simulink model "experiment"  (R2021b)
settings: Solver=VariableStepAuto  StartTime=0.0  StopTime=40  FixedStep=1  RelTol=1e-3
InitFcn:
  | InitFcn;
StopFcn:
  | PostFunction;
values from neighbouring files (symbols this model uses):
  desiredSpeed = -10    [InitFcn.m]
  LookDistance = 0.4    [InitFcn.m]
  vehicleDynamics = [b1 L1 L2 b2]    [InitFcn.m]
  X_waypoints = [X_waypoints, linspace(L1-L2-R1, L1-L2-R1, n)]    [InitFcn.m]
  Y_waypoints = [Y_waypoints, linspace(-R1,-R1-L3,n)]    [InitFcn.m]
undefined symbols (not defined in the file or in its folder): Index, X_waypoints_2, Y_waypoints_2
libraries: slpidlib x1
settings Model: Creator=juliu  LastModifiedBy=marti
settings SolverCC: AlgebraicLoopSolver=TrustRegion
settings DataIOCC: SaveFormat=StructureWithTime  ReturnWorkspaceOutputs=off
settings OptimizationCC: BlockReduction=off  BufferReuse=off
settings DebuggingCC: AlgebraicLoopMsg=none  UnconnectedInputMsg=none  UnconnectedOutputMsg=none  UnconnectedLineMsg=none  SFMachineParentedDataDiag=warning

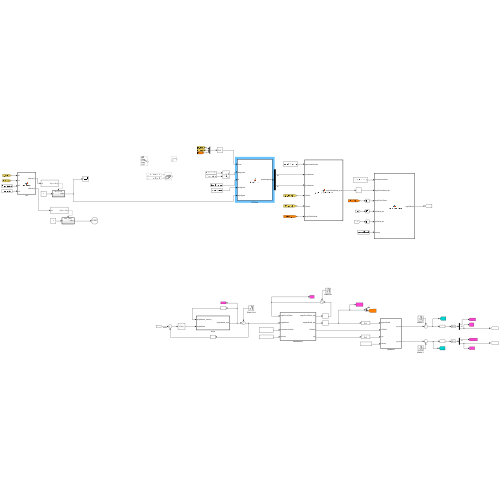
[thumbnail: Simulink's stored preview of the top-level diagram]
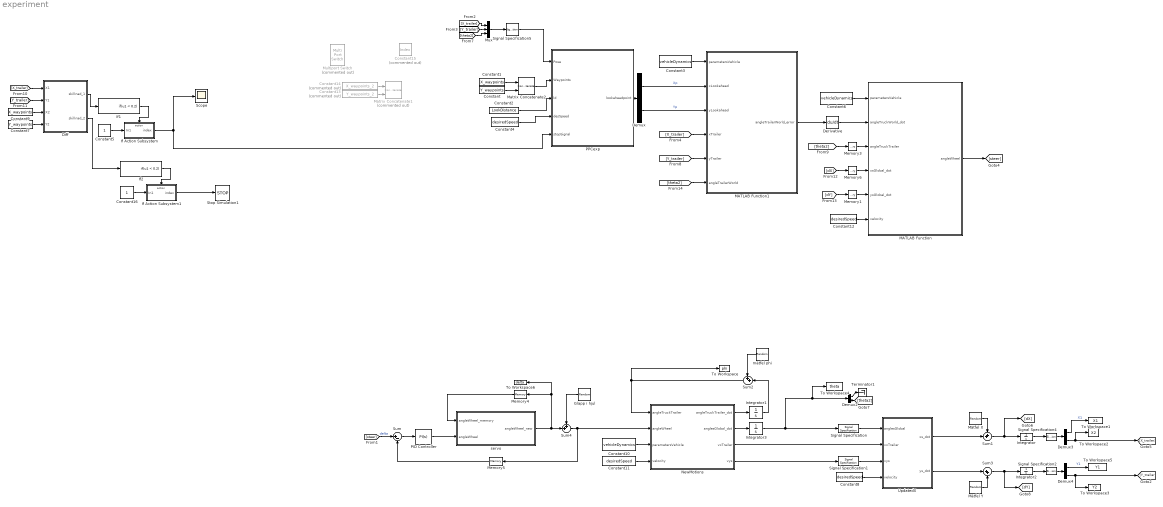
== system experiment ==
  Constant : Constant  Value=Y_waypoints
  Constant1 : Constant  Value=X_waypoints
  Constant10 : Constant  Value=vehicleDynamics
  Constant{4,8,11..12} (4 alike) : Constant  Value=desiredSpeed
  Constant13 : Constant  Commented=on  Value=Y_waypoints_2
  Constant14 : Constant  Commented=on  Value=X_waypoints_2
  Constant15 : Constant  Commented=on  Value=Index
  Constant16 : Constant
  Constant2 : Constant  Value=LookDistance
  Constant3 : Constant  Value=vehicleDynamics
  Constant5 : Constant
  Constant6 : Constant  Value=vehicleDynamics
  Constant7 : Constant  Value=Y_waypoints
  Constant9 : Constant  Value=X_waypoints
  Demux{,2..4} (4 alike) : Demux  Outputs=2
  Derivative : Derivative
  Diff : MATLAB Function  TreatAsAtomicUnit=on
  Glapp i hjul : RandomNumber  Variance=(pi/360)^2  SampleTime=3
  If Action Subsystem : Subsystem  TreatAsAtomicUnit=on
  If Action Subsystem1 : Subsystem  TreatAsAtomicUnit=on
  If1 : If  IfExpression=u1 < 0.2  ShowElse=off
  If2 : If  IfExpression=u1 < 0.2  ShowElse=off
  Integrator : Integrator  InitialCondition=[0;-1.3]
  Integrator1 : Integrator
  Integrator2 : Integrator
  Integrator3 : Integrator
  MATLAB Function : MATLAB Function  TreatAsAtomicUnit=on
  MATLAB Function1 : MATLAB Function  TreatAsAtomicUnit=on
  Matrix Concatenate1 : Concatenate  Commented=on  Mode=Multidimensional array  ConcatenateDimension=2
  Matrix Concatenate2 : Concatenate  Mode=Multidimensional array  ConcatenateDimension=2
  Memory{1,3..6} (5 alike) : Memory
  Multiport Switch : MultiPortSwitch  Commented=on
  Mux : Mux  Inputs=3
  Mätfel X : RandomNumber  Variance=(4e-5)^2  SampleTime=0.1
  Mätfel Y : RandomNumber  Variance=(4e-5)^2  SampleTime=0.1
  NewMotions : MATLAB Function  TreatAsAtomicUnit=on
  PID Controller : slpidlib/PID Controller  Controller=PI  Form=Parallel  TimeDomain=Continuous-time  UseExternalTs=off  SampleTime=-1  IntegratorMethod=Forward Euler  FilterMethod=Forward Euler  ControllerParametersSource=internal  P=2.10  I=0.50  D=0  UseFilter=on  N=100  TunerSelectOption=Transfer Function Based (PID Tuner App)  InitialConditionSource=internal  InitialConditionForIntegrator=0  InitialConditionForFilter=0  DifferentiatorICPrevScaledInput=0  ExternalReset=none  TrackingMode=off  Kt=1  LimitOutput=off  SatLimitsSource=internal  UpperSaturationLimit=inf  LowerSaturationLimit=-inf  LinearizeAsGain=on  AntiWindupMode=none  Kb=1  POutMin=[]  POutMax=[]  IOutMin=[]  IOutMax=[]  DOutMin=[]  DOutMax=[]  NOutMin=[]  NOutMax=[]  SumOutMin=[]  SumOutMax=[]  SaturationOutMin=[]  SaturationOutMax=[]  PParamMin=[]  PParamMax=[]  IParamMin=[]  IParamMax=[]  DParamMin=[]  DParamMax=[]  NParamMin=[]  NParamMax=[]  KbParamMin=[]  KbParamMax=[]  KtParamMin=[]  KtParamMax=[]  KbOutMin=[]  KbOutMax=[]  KtOutMin=[]  KtOutMax=[]  IntegratorOutMin=[]  IntegratorOutMax=[]  FilterOutMin=[]  FilterOutMax=[]  SumI1OutMin=[]  SumI1OutMax=[]  SumI2OutMin=[]  SumI2OutMax=[]  SumI3OutMin=[]  SumI3OutMax=[]  SumI4OutMin=[]  SumI4OutMax=[]  SumDOutMin=[]  SumDOutMax=[]  DifferentiatorOutMin=[]  DifferentiatorOutMax=[]  FilterDiffOutCoefMin=[]  FilterDiffOutCoefMax=[]  ReciprocalOutMin=[]  ReciprocalOutMax=[]  SumDenOutMin=[]  SumDenOutMax=[]  SumNumOutMin=[]  SumNumOutMax=[]  DivideOutMin=[]  DivideOutMax=[]  UdiffTsProdOutMin=[]  UdiffTsProdOutMax=[]  NTsProdOutMin=[]  NTsProdOutMax=[]  UintegralTsProdOutMin=[]  UintegralTsProdOutMax=[]  UngainTsProdOutMin=[]  UngainTsProdOutMax=[]  IntegratorContinuousStateAttributes=''  IntegratorStateMustResolveToSignalObject=off  IntegratorRTWStateStorageClass=Auto  FilterContinuousStateAttributes=''  FilterStateMustResolveToSignalObject=off  FilterRTWStateStorageClass=Auto  ParallelPVariant=InternalParameters  IdealPVariant=Disabled  IVariant=InternalParameters  DVariant=Disabled  IntegratorVariant=Continuous  SatVariant=Disabled  AWVariant=Passthrough  PCopyVariant=Disabled  TRVariant=Disabled  FdbkBlocksVariant=Forward  IdealPFdbkVariant=Disabled  SatFdbkVariant=Disabled  DerivativeFilterVariant=Disabled  NVariant=Disabled  NCopyVariant=Disabled_SignalSpec  FilterICVariant=Disabled  IntegratorICVariant=InternalICs  ExternalResetVariant=Disabled  TRSumVariant=Passthrough  SumFdbkVariant=Disabled  SumVariant=Sum_PI  TsampFilterVariant=InternalTs  TsampNgainVariant=Passthrough  TsampIntegralVariant=Passthrough  ExternalSaturationOutDataTypeStr=Inherit: Same as second input
  PPCexp : MATLAB Function  TreatAsAtomicUnit=on
  Scope : Scope
  Signal Specification{,1..2,4} (4 alike) : SignalSpecification  Dimensions=2
  Signal Specification5 : SignalSpecification  Dimensions=3
  Stop Simulation1 : Stop
  Sum : Sum  Inputs=|+-
  Sum1 : Sum  Inputs=++|
  Sum2 : Sum  Inputs=++|
  Sum3 : Sum  Inputs=|++
  Sum4 : Sum  Inputs=++|
  Terminator1 : Terminator
  To Workspace : ToWorkspace  VariableName=phi  SampleTime=-1
  To Workspace1 : ToWorkspace  VariableName=X1  SampleTime=-1
  To Workspace2 : ToWorkspace  VariableName=X2  SampleTime=-1
  To Workspace3 : ToWorkspace  VariableName=Y2  SampleTime=-1
  To Workspace4 : ToWorkspace  VariableName=theta  SampleTime=-1
  To Workspace5 : ToWorkspace  VariableName=Y1  SampleTime=-1
  To Workspace6 : ToWorkspace  VariableName=delta  SampleTime=-1
  UpdatedX : MATLAB Function  TreatAsAtomicUnit=on
  mätfel phi : RandomNumber  Variance=(pi/360)^2  SampleTime=0.01
  servo : MATLAB Function  TreatAsAtomicUnit=on
  wires:
  Demux/1 -> MATLAB Function1/2(xLookahead)  "Xp"
  PPCexp/1(lookaheadpoint) -> Demux/1
  NewMotions/3(vxTrailer) -> UpdatedX/2(vxTrailer)
  Mux/1 -> Signal Specification5/1
  [Y_trailer] -> Mux/2
  [X_trailer] -> Mux/1
  Constant1/1 -> Matrix Concatenate2/1
  Constant/1 -> Matrix Concatenate2/2
  Constant2/1 -> PPCexp/3(ld)
  Integrator2/1 -> Signal Specification2/1
  Integrator/1 -> Signal Specification4/1
  NewMotions/1(angleTruckTrailer_dot) -> Integrator1/1
  NewMotions/2(anglesGlobal_dot) -> Integrator3/1
  Integrator3/1 -> Signal Specification/1, Demux2/1, To Workspace4/1
  Demux2/1 -> Terminator1/1
  Constant8/1 -> UpdatedX/4(velocity)
  Signal Specification/1 -> UpdatedX/1(anglesGlobal)
  NewMotions/4(vys) -> Signal Specification1/1
  Signal Specification1/1 -> UpdatedX/3(vys)
  Signal Specification2/1 -> Demux4/1
  Demux3/1 -> To Workspace1/1  "X1"
  Demux4/1 -> To Workspace5/1  "Y1"
  Demux3/2 -> To Workspace2/1, [X_trailer]
  [theta2] -> Mux/3
  Derivative/1 -> MATLAB Function/2(angleTruckWorld_dot)
  [X_trailer] -> MATLAB Function1/4(xTrailer)
  [Y_trailer] -> MATLAB Function1/5(yTrailer)
  MATLAB Function/1(angleWheel) -> [steer]
  Memory3/1 -> MATLAB Function/3(angleTruckTrailer)
  MATLAB Function1/1(angleTrailerWorld_error) -> Derivative/1
  Signal Specification4/1 -> Demux3/1
  [theta2] -> MATLAB Function1/6(angleTrailerWorld)
  Demux2/2 -> [theta2]
  Integrator1/1 -> Sum2/2
  Sum2/1 -> To Workspace/1, NewMotions/1(angleTruckTrailer)
  Mätfel X/1 -> Sum1/1
  UpdatedX/1(xs_dot) -> Sum1/2
  Sum1/1 -> [dX], Integrator/1
  Sum3/1 -> [dY], Integrator2/1
  mätfel phi/1 -> Sum2/1
  [theta2] -> Memory3/1
  servo/1(angleWheel_new) -> To Workspace6/1, Memory4/1, Sum4/2
  Memory4/1 -> servo/1(angleWheel_memory)
  PID Controller/1 -> servo/2(angleWheel)
  [steer] -> Sum/1  "delta"
  Sum/1 -> PID Controller/1
  Sum4/1 -> Memory5/1, NewMotions/2(angleWheel)
  Memory5/1 -> Sum/2
  Demux/2 -> MATLAB Function1/3(yLookahead)  "Yp"
  Constant9/1 -> Diff/3(X2)
  Constant7/1 -> Diff/4(Y2)
  [Y_trailer] -> Diff/2(Y1)
  [X_trailer] -> Diff/1(X1)
  Diff/1(skillnad_1) -> If1/1
  If1/1 -> If Action Subsystem/Action
  Constant5/1 -> If Action Subsystem/1(In1)
  Mätfel Y/1 -> Sum3/2
  UpdatedX/2(ys_dot) -> Sum3/1
  Memory6/1 -> MATLAB Function/4(xsGlobal_dot)
  Memory1/1 -> MATLAB Function/5(ysGlobal_dot)
  [dX] -> Memory6/1
  [dY] -> Memory1/1
  Constant3/1 -> MATLAB Function1/1(parametersVehicle)
  Constant6/1 -> MATLAB Function/1(parametersVehicle)
  Constant10/1 -> NewMotions/3(parametersVehicle)
  Constant11/1 -> NewMotions/4(velocity)
  Constant12/1 -> MATLAB Function/6(velocity)
  Demux4/2 -> To Workspace3/1, [Y_trailer]
  Glapp i hjul/1 -> Sum4/1
  Constant13/1 -> Matrix Concatenate1/2
  Constant14/1 -> Matrix Concatenate1/1
  If Action Subsystem/1(index) -> Scope/1, PPCexp/5(stopSignal)
  Signal Specification5/1 -> PPCexp/1(Pose)
  Matrix Concatenate2/1 -> PPCexp/2(Waypoints)
  Constant4/1 -> PPCexp/4(desSpeed)
  Diff/2(skillnad_2) -> If2/1
  If Action Subsystem1/1(index) -> Stop Simulation1/1
  Constant16/1 -> If Action Subsystem1/1(In1)
  If2/1 -> If Action Subsystem1/Action

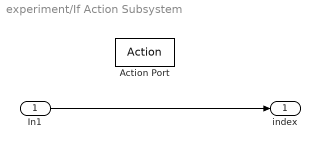
== system experiment/If Action Subsystem ==
  In1 : Inport
  Action Port : ActionPort  ActionPortLabel=if(u1 < 0.2)
  index : Outport
  wires:
  In1/1 -> index/1

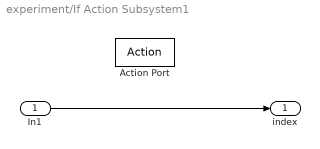
== system experiment/If Action Subsystem1 ==
  In1 : Inport
  Action Port : ActionPort  ActionPortLabel=if(u1 < 0.2)
  index : Outport
  wires:
  In1/1 -> index/1

== matlab function experiment/servo ==
  data: angleWheel_memory input; angleWheel input; angleWheel_new output
function angleWheel_new = MotorAngle(angleWheel_memory, angleWheel)
    rotationThreshold = pi/180;
    
    rotation = angleWheel - angleWheel_memory;
    if abs(rotation) > rotationThreshold
        angleWheel_new = angleWheel_memory + sign(rotation) * rotationThreshold;
    else
        angleWheel_new = angleWheel;
    end

    angleWheel_new = min(max(angleWheel_new, -pi * 28 / 180), pi * 28 / 180); % clamp(num, min bound, max bound)
end

== matlab function experiment/PPCexp ==
  data: Pose input; Waypoints input; ld input; desSpeed input; lookaheadpoint output; stopSignal input
function lookaheadpoint = PurePursuit(Pose, Waypoints, ld, desSpeed, stopSignal)

% ORGINAL
%controller = controllerPurePursuit('DesiredLinearVelocity', abs(desSpeed), 'Waypoints', Waypoints, 'LookaheadDistance',ld); 

% FÖRSTA HÄLFTEN
%controller = controllerPurePursuit('DesiredLinearVelocity', abs(desSpeed), 'Waypoints', Waypoints(1:end/2,:), 'LookaheadDistance',ld);

if(stopSignal <= 0.5)
    controller = controllerPurePursuit('DesiredLinearVelocity', abs(desSpeed), 'Waypoints', Waypoints(1:end/2,:), 'LookaheadDistance',ld);
else
    controller = controllerPurePursuit('DesiredLinearVelocity', abs(desSpeed), 'Waypoints', Waypoints(end/2:end,:), 'LookaheadDistance',ld);
end

[vel,angvel,lookaheadpoint] = controller(Pose);% pose is the orientation of vehicle

== matlab function experiment/NewMotions ==
  data: angleTruckTrailer input; angleTruckTrailer_dot output; angleWheel input; parametersVehicle input; anglesGlobal_dot output; vxTrailer output; vys output; velocity input
%This function is our "Plant" in here is all the kinematics of trailer and
%dolly. It output is change in phi and theta and velocity in x and y
%direction. Most of this is taken from the previous code but change in
%varibale names
function [angleTruckTrailer_dot, anglesGlobal_dot, vxTrailer, vys] = Motions(angleTruckTrailer, angleWheel, parametersVehicle, velocity)
    b_d = parametersVehicle(1); % Length from rear-axle to center of dolly
    L_d = parametersVehicle(2); % Length of between wheels dolly
    L_s = parametersVehicle(3); % Length between wheelbase and connection of trailer
    b_s = parametersVehicle(4); % Trailer slip of

    angleTruckTrailer_dot = 0;         % Hitch angle at point A    
    anglesGlobal_dot = [0;0];     % Change in yaw angles

    vxTrailer = 0;           % Longitudinal velocity
    vys=[0;0];

    %dolly
    anglesGlobal_dot(1) = (velocity / L_d) * tan(angleWheel); %yaw rate of the tractor [rad/s]
    vys(1) = b_d * anglesGlobal_dot(1);       % Lateral velocity at point A

    %släp
    anglesGlobal_dot(2) =(1 / L_s) * (-velocity * sin(angleTruckTrailer) + cos(angleTruckTrailer) * vys(1)); %Yaw rate of trailer 1 [rad/s]
    vxTrailer = velocity * cos(angleTruckTrailer) + vys(1) * sin(angleTruckTrailer); % longitudinal velocity at point B
    vys(2) = -anglesGlobal_dot(2) * b_s; % Lateral velocity at point B
    angleTruckTrailer_dot = anglesGlobal_dot(2) - anglesGlobal_dot(1); %Articulation angle rate at pivot 1 [rad/s]
end

== matlab function experiment/UpdatedX ==
  data: anglesGlobal input; xs_dot output; vxTrailer input; vys input; velocity input; ys_dot output
function [xs_dot, ys_dot] = GlobalPos(anglesGlobal, vxTrailer, vys, velocity)
    xs_dot=[0;0];
    xs_dot(1) = velocity*cos(anglesGlobal(1))-vys(1)*sin(anglesGlobal(1));
    xs_dot(2) = vxTrailer*cos(anglesGlobal(2))-vys(2)*sin(anglesGlobal(2));

    ys_dot=[0;0];
    ys_dot(1) = vys(1)*cos(anglesGlobal(1))+velocity*sin(anglesGlobal(1));
    ys_dot(2) = vys(2)*cos(anglesGlobal(2))+vxTrailer*sin(anglesGlobal(2));  
end

== matlab function experiment/Diff ==
  data: X1 input; skillnad_1 output; Y1 input; X2 input; Y2 input; skillnad_2 output
function [skillnad_1, skillnad_2]    = diffunktion(X1,Y1,X2,Y2)
trailer=[X1 Y1];
path_1=[X2(end/2) Y2(end/2)];
path_2=[X2(end) Y2(end)];
skillnad_1 = norm(path_1-trailer);
skillnad_2 = norm(path_2-trailer);

%Index = 2;
end

== matlab function experiment/MATLAB Function ==
  data: parametersVehicle input; angleTruckWorld_dot input; angleWheel output; angleTruckTrailer input; xsGlobal_dot input; ysGlobal_dot input; velocity input
%This function is supposed to calculate a desired steeringangle so that
%phi_des is meet. 

function angleWheel = UpdateWheelAngle(parametersVehicle, angleTruckWorld_dot, angleTruckTrailer, xsGlobal_dot, ysGlobal_dot, velocity)
    b_d = parametersVehicle(1);
    L_d = parametersVehicle(2);
    L_s = parametersVehicle(3);
    b_s = parametersVehicle(4);

    dtheta2 = (xsGlobal_dot(1) * sin(angleTruckTrailer) - ysGlobal_dot(1) * cos(angleTruckTrailer)) / L_s;
    angleWheel = -atan((dtheta2 - angleTruckWorld_dot) * L_d / velocity);
end

== matlab function experiment/MATLAB Function1 ==
  data: parametersVehicle input; angleTrailerWorld_error output; xLookahead input; yLookahead input; xTrailer input; yTrailer input; angleTrailerWorld input
%this funciton calculates phi_error which is the diffrence of angle between
%theta (trailers position angle) and the lookahead point (desired heading 
%angle). Which gives us phi_des, desired angle between trailer and dolly

function angleTrailerWorld_error = UpdateTrailerWorldAngle(parametersVehicle, xLookahead, yLookahead, xTrailer, yTrailer, angleTrailerWorld)
    b_d = parametersVehicle(1);
    L_d = parametersVehicle(2);
    L_s = parametersVehicle(3);
    b_s = parametersVehicle(4);

    deltaX = xTrailer - xLookahead;
    deltaY = yTrailer - yLookahead;

    XY_diff = sqrt(deltaX^2 + deltaY^2);

    % Använd atan2(deltaY / deltaX) - theta2? Löser detta...
    theta2_err = acos(deltaX / XY_diff) - angleTrailerWorld;
    if deltaY<0     %för att den ska gå varvet runt, klarar dock bara 3/4,verkar bero på waypoints
        theta2_err = pi + acos(-deltaX / XY_diff) - angleTrailerWorld;
    end
    
    angleTrailerWorld_error = -3 * atan2(2 * L_s * sin(theta2_err), XY_diff);
end
